simulink model "acc_aeb"  (R2024b)
settings: Solver=FixedStepDiscrete  StartTime=0.0  StopTime=60  FixedStep=0.02  RelTol=1e-3
model workspace (MAT data in the model file):
  memory_initial = [0; 0; 5.5555555556; 0]
  scenario_input = [0 0.02 0.04 0.06 0.08 0.1 0.12 0.14 0.16 0.18 0.2 0.22 ... (12004 elements, 3001x4)]
  vehicle_initial = [22.2222222222; 22.2222222222; 45; 0]
(part 1 of 2)
settings Model: Creator=runner  LastModifiedBy=runner

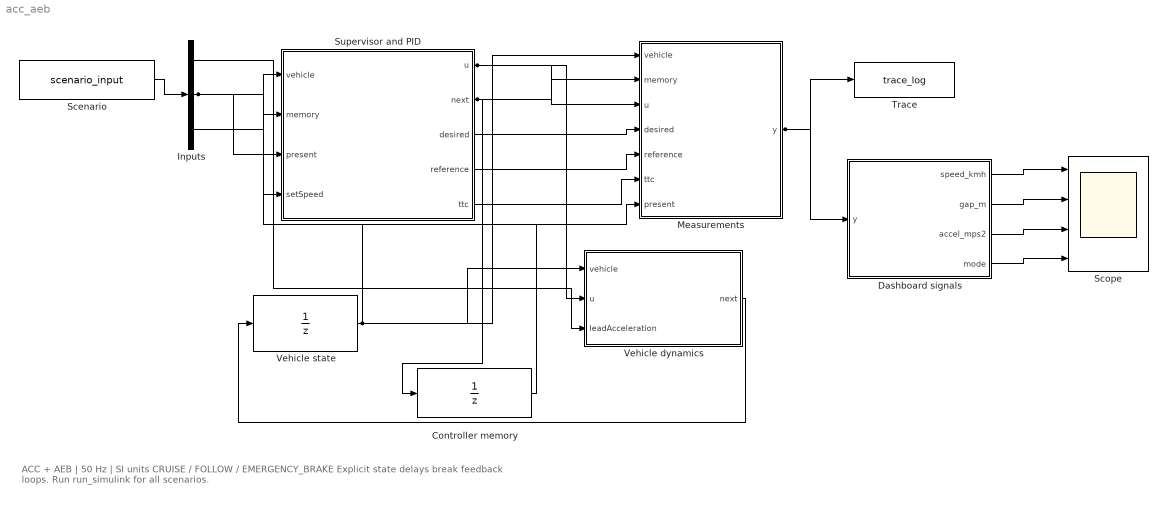
== system acc_aeb ==
  note: ACC + AEB | 50 Hz | SI units
      | CRUISE / FOLLOW / EMERGENCY_BRAKE
      | Explicit state delays break feedback loops. Run run_simulink for all scenarios.
  Controller memory : UnitDelay  InitialCondition=memory_initial  SampleTime=0.02  HasFrameUpgradeWarning=on
  Dashboard signals : MATLAB Function  TreatAsAtomicUnit=on
  Inputs : Demux  Outputs=3
  Measurements : MATLAB Function  TreatAsAtomicUnit=on
  Scenario : FromWorkspace  VariableName=scenario_input  SampleTime=0.02  Interpolate=off  OutputAfterFinalValue=Holding final value
  Scope : Scope  NumInputPorts=4
  Supervisor and PID : MATLAB Function  TreatAsAtomicUnit=on
  Trace : ToWorkspace  VariableName=trace_log  SaveFormat=Structure With Time  SampleTime=-1
  Vehicle dynamics : MATLAB Function  TreatAsAtomicUnit=on
  Vehicle state : UnitDelay  InitialCondition=vehicle_initial  SampleTime=0.02  HasFrameUpgradeWarning=on
  wires:
  Scenario/1 -> Inputs/1
  Inputs/1 -> Vehicle dynamics/3(leadAcceleration)
  Inputs/2 -> Supervisor and PID/3(present), Measurements/7(present)
  Inputs/3 -> Supervisor and PID/4(setSpeed)
  Vehicle state/1 -> Supervisor and PID/1(vehicle), Vehicle dynamics/1(vehicle), Measurements/1(vehicle)
  Controller memory/1 -> Supervisor and PID/2(memory)
  Supervisor and PID/1(u) -> Vehicle dynamics/2(u), Measurements/3(u)
  Supervisor and PID/2(next) -> Controller memory/1, Measurements/2(memory)
  Supervisor and PID/3(desired) -> Measurements/4(desired)
  Supervisor and PID/4(reference) -> Measurements/5(reference)
  Supervisor and PID/5(ttc) -> Measurements/6(ttc)
  Vehicle dynamics/1(next) -> Vehicle state/1
  Measurements/1(y) -> Trace/1, Dashboard signals/1(y)
  Dashboard signals/1(speed_kmh) -> Scope/1
  Dashboard signals/2(gap_m) -> Scope/2
  Dashboard signals/3(accel_mps2) -> Scope/3
  Dashboard signals/4(mode) -> Scope/4
